simulink model "kompfilter"  (R2023a)
settings: Solver=VariableStepAuto  StartTime=0.0  StopTime=tend  RelTol=1e-3
libraries: cstblocks x6
settings Model: Creator=Xenjamo  LastModifiedBy=Xenjamo

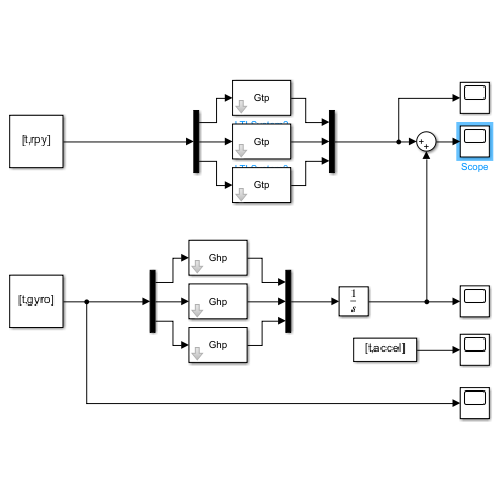
[thumbnail: Simulink's stored preview of the top-level diagram]
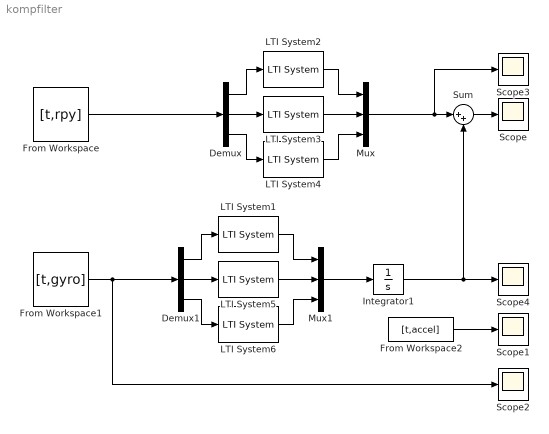
== system kompfilter ==
  Demux : Demux  Outputs=3
  Demux1 : Demux  Outputs=3
  From Workspace : FromWorkspace  VariableName=[t,rpy]
  From Workspace1 : FromWorkspace  VariableName=[t,gyro]
  From Workspace2 : FromWorkspace  VariableName=[t,accel]
  Integrator1 : Integrator
  LTI System1 : cstblocks/LTI System  sys=Ghp  IC=[]
  LTI System2 : cstblocks/LTI System  sys=Gtp  IC=[]
  LTI System3 : cstblocks/LTI System  sys=Gtp  IC=[]
  LTI System4 : cstblocks/LTI System  sys=Gtp  IC=[]
  LTI System5 : cstblocks/LTI System  sys=Ghp  IC=[]
  LTI System6 : cstblocks/LTI System  sys=Ghp  IC=[]
  Mux : Mux  Inputs=3
  Mux1 : Mux  Inputs=3
  Scope{,1..4} (5 alike) : Scope
  Sum : Sum  Inputs=|++
  wires:
  From Workspace1/1 -> Demux1/1, Scope2/1
  Mux/1 -> Scope3/1, Sum/1
  Sum/1 -> Scope/1
  From Workspace/1 -> Demux/1
  Demux/1 -> LTI System2/1
  Demux/2 -> LTI System3/1
  Demux/3 -> LTI System4/1
  LTI System2/1 -> Mux/1
  LTI System3/1 -> Mux/2
  LTI System4/1 -> Mux/3
  Mux1/1 -> Integrator1/1
  Demux1/1 -> LTI System1/1
  Demux1/2 -> LTI System5/1
  LTI System6/1 -> Mux1/3
  Demux1/3 -> LTI System6/1
  From Workspace2/1 -> Scope1/1
  LTI System5/1 -> Mux1/2
  LTI System1/1 -> Mux1/1
  Integrator1/1 -> Sum/2, Scope4/1
